simulink model "sanduan"  (R2018b)
settings: Solver=ode23s  StartTime=0.0  StopTime=2  RelTol=1e-3
libraries: powerlib_meascontrol x27, simulink_extras x27, powerlib x13
settings Model: Creator=snial  LastModifiedBy=snailtiny
settings DataIOCC: SaveFormat=StructureWithTime
settings OptimizationCC: LifeSpan=inf
settings DebuggingCC: SFExecutionAtInitializationDiag=none
settings HardwareCC: ProdBitPerSizeT=32  ProdBitPerPtrDiffT=32  ProdWordSize=32  ProdHWDeviceType=Specified
settings SFSimCC: SimUseLocalCustomCode=off
settings RTWCC: RTWUseLocalCustomCode=off
settings CodeAppCC: StateflowObjectComments=on
settings SimscapeCC: SimscapeNormalizeSystem=off

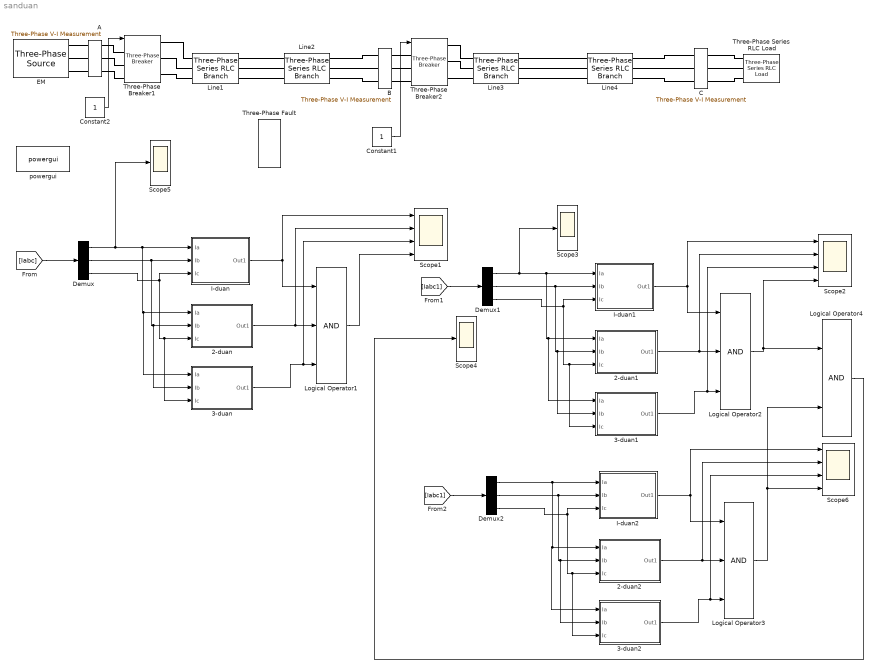
== system sanduan ==
  2-duan : Subsystem
  2-duan1 : Subsystem
  2-duan2 : Subsystem
  3-duan : Subsystem
  3-duan1 : Subsystem
  3-duan2 : Subsystem
  A : powerlib/Measurements/Three-Phase V-I Measurement  VoltageMeasurement=phase-to-ground  SetLabelV=on  LabelV=Vabc  Vpu=off  VpuLL=off  CurrentMeasurement=yes  SetLabelI=on  LabelI=Iabc  Ipu=off  Pbase=100e6  Vbase=500e3  OutputType=Complex  PhasorSimulation=off  PSBequivalent=0
      settings: SourceProductName=Simscape Electrical
  B : powerlib/Measurements/Three-Phase V-I Measurement  VoltageMeasurement=phase-to-ground  SetLabelV=on  LabelV=Vabc1  Vpu=off  VpuLL=off  CurrentMeasurement=yes  SetLabelI=on  LabelI=Iabc1  Ipu=off  Pbase=100e6  Vbase=500e3  OutputType=Complex  PhasorSimulation=off  PSBequivalent=0
      settings: SourceProductName=Simscape Electrical
  C : powerlib/Measurements/Three-Phase V-I Measurement  VoltageMeasurement=phase-to-ground  SetLabelV=on  LabelV=Vabc2  Vpu=off  VpuLL=off  CurrentMeasurement=yes  SetLabelI=on  LabelI=Iabc2  Ipu=off  Pbase=100e6  Vbase=500e3  OutputType=Complex  PhasorSimulation=off  PSBequivalent=0
      settings: SourceProductName=Simscape Electrical
  Constant1 : Constant
  Constant2 : Constant
  Demux : Demux  Outputs=3
  Demux1 : Demux  Outputs=3
  Demux2 : Demux  Outputs=3
  EM : powerlib/Electrical Sources/Three-Phase Source  InternalConnection=Yg  VoltagePhases=off  Voltage=37e3  PhaseAngle=0  Voltage_phases=[25e3 25e3 25e3]/sqrt(3)  PhaseAngles_phases=[0 -120 +120]  Frequency=50  NonIdealSource=on  SpecifyImpedance=off  Resistance=6  Inductance=0  ShortCircuitLevel=100e6  BaseVoltage=37e3  XRratio=7  BusType=swing  Pref=10e3  Qref=0  Prefabc=[10e3, 10e3, 10e3]  Qrefabc=[0, 0, 0]  Qmin=-inf  Qmax=inf
      settings: SourceProductName=Simscape Electrical
  I-duan : Subsystem
  I-duan1 : Subsystem
  I-duan2 : Subsystem
  Line1 : powerlib/Elements/Three-Phase Series RLC Branch  LConnTagsString=A|B|C  RConnTagsString=A|B|C  BranchType=R  Resistance=2  Inductance=0.00318*2  Capacitance=1e-6  Measurements=None
      settings: SourceProductName=Simscape Electrical
  Line2 : powerlib/Elements/Three-Phase Series RLC Branch  LConnTagsString=A|B|C  RConnTagsString=A|B|C  BranchType=R  Resistance=8  Inductance=0.00318*8  Capacitance=1e-6  Measurements=None
      settings: SourceProductName=Simscape Electrical
  Line3 : powerlib/Elements/Three-Phase Series RLC Branch  LConnTagsString=A|B|C  RConnTagsString=A|B|C  BranchType=R  Resistance=2  Inductance=0.00318*24  Capacitance=1e-6  Measurements=None
      settings: SourceProductName=Simscape Electrical
  Line4 : powerlib/Elements/Three-Phase Series RLC Branch  LConnTagsString=A|B|C  RConnTagsString=A|B|C  BranchType=R  Resistance=14  Inductance=0.00318*24  Capacitance=1e-6  Measurements=None
      settings: SourceProductName=Simscape Electrical
  Logical Operator1 : Logic  Inputs=3  AllPortsSameDT=off  OutDataTypeStr=boolean
  Logical Operator2 : Logic  Inputs=3  AllPortsSameDT=off  OutDataTypeStr=boolean
  Logical Operator3 : Logic  Inputs=3  AllPortsSameDT=off  OutDataTypeStr=boolean
  Logical Operator4 : Logic  AllPortsSameDT=off  OutDataTypeStr=boolean
  Scope1 : Scope  NumInputPorts=4
  Scope2 : Scope  NumInputPorts=4
  Scope3 : Scope
  Scope4 : Scope
  Scope5 : Scope
  Scope6 : Scope  NumInputPorts=4
  Three-Phase Series RLC Load : powerlib/Elements/Three-Phase Series RLC Load  LConnTagsString=A|B|C  Configuration=Y (grounded)  NominalVoltage=37e3  Vabc=[1e3 1e3 1e3]  Vabcp=[1e3 1e3 1e3]  NominalFrequency=50  UnbalancedPower=off  ActivePower=6.4e6  InductivePower=0  CapacitivePower=0  Pabc=[10e3 9e3 11e3]  QLabc=[100 90 110]  QCabc=[100 90 110]  Pabcp=[10e3 9e3 11e3]  QLabcp=[100 90 110]  QCabcp=[100 90 110]  Measurements=None  LoadType=constant Z
      settings: SourceProductName=Simscape Electrical
  Three-Phase Breaker1 : powerlib/Elements/Three-Phase Breaker  InitialState=closed  SwitchA=on  SwitchB=on  SwitchC=on  SwitchTimes="[1  1.20]"  External=on  BreakerResistance=0.0000000000000000001  SnubberResistance=1e6  SnubberCapacitance=inf  Measurements=None
      settings: SourceProductName=Simscape Electrical
  Three-Phase Breaker2 : powerlib/Elements/Three-Phase Breaker  InitialState=closed  SwitchA=on  SwitchB=on  SwitchC=on  SwitchTimes="[1  1.20]"  External=on  BreakerResistance=0.0000000000000000001  SnubberResistance=1e6  SnubberCapacitance=inf  Measurements=None
      settings: SourceProductName=Simscape Electrical
  Three-Phase Fault : powerlib/Elements/Three-Phase Fault  InitialStates=0  FaultA=on  FaultB=on  FaultC=off  GroundFault=off  SwitchTimes=[0.2 0.5]  External=off  SwitchStatus=NaN  FaultResistance=20  GroundResistance=0.01  SnubberResistance=inf  SnubberCapacitance=0  Measurements=None
      settings: SourceProductName=Simscape Electrical
  powergui : powerlib/powergui  Priority=1  SimulationMode=Continuous  SampleTime=1e-10  frequency=50  Iterations=50  frequencyindice=50  Pbase=100e6  ErrMax=1e-4  UnitsV=kV  UnitsW=MW  buscounter=0  FunctionMessages=off  echomessages=off  EnableUseOfTLC=off  CurrentSourceSwitches=off  DisableSnubberDevices=off  DisableRonSwitches=off  DisableVfSwitches=off  DisplayEquations=off  SolverType=Tustin/Backward Euler (TBE)  Interpol=off  ExternalGateDelay=off  methode=off  Ts=100  x0status=blocks  SPID=on  SwTol=0  HookPort=off  RestoreLinks=warning  ResistiveCurrentMeasurement=off  Frange=[0:2:500]  Ylog=off  Xlog=on  ShowGrid=off  save=off  variable=ZData  structure=0  ZoomFFT=off  StartTime=0.0  cycles=1  DisplayStyle=1  fundamental=60  FreqAxis=off  MaxFrequency=1000  frequencyindicesteady=1  RmsSteady=1  display=off
  wires:
  [Iabc] -> Demux/1
  Demux/1 -> Scope5/1, 3-duan/1(Ia), 2-duan/1(Ia), I-duan/1(Ia)
  Demux/2 -> 3-duan/2(Ib), 2-duan/2(Ib), I-duan/2(Ib)
  Demux/3 -> 3-duan/3(Ic), 2-duan/3(Ic), I-duan/3(Ic)
  I-duan/1(Out1) -> Scope1/1, Logical Operator1/1
  2-duan/1(Out1) -> Scope1/2, Logical Operator1/2
  3-duan/1(Out1) -> Scope1/3, Logical Operator1/3
  Logical Operator1/1 -> Scope1/4
  [Iabc1] -> Demux1/1
  Demux1/1 -> Scope3/1, 3-duan1/1(Ia), 2-duan1/1(Ia), I-duan1/1(Ia)
  Demux1/2 -> 3-duan1/2(Ib), 2-duan1/2(Ib), I-duan1/2(Ib)
  Demux1/3 -> 3-duan1/3(Ic), 2-duan1/3(Ic), I-duan1/3(Ic)
  I-duan1/1(Out1) -> Logical Operator2/1, Scope2/1
  2-duan1/1(Out1) -> Scope2/2, Logical Operator2/2
  3-duan1/1(Out1) -> Scope2/3, Logical Operator2/3
  Logical Operator2/1 -> Scope2/4, Logical Operator4/1
  Demux2/3 -> 3-duan2/3(Ic), 2-duan2/3(Ic), I-duan2/3(Ic)
  2-duan2/1(Out1) -> Scope6/2, Logical Operator3/2
  I-duan2/1(Out1) -> Scope6/1, Logical Operator3/1
  [Iabc1] -> Demux2/1
  Logical Operator3/1 -> Logical Operator4/2, Scope6/4
  Demux2/1 -> 3-duan2/1(Ia), 2-duan2/1(Ia), I-duan2/1(Ia)
  3-duan2/1(Out1) -> Scope6/3, Logical Operator3/3
  Demux2/2 -> 3-duan2/2(Ib), 2-duan2/2(Ib), I-duan2/2(Ib)
  Logical Operator4/1 -> Scope4/1
  Constant2/1 -> Three-Phase Breaker1/1
  Constant1/1 -> Three-Phase Breaker2/1
  connections:
  A/LConn1 -- EM/RConn1
  A/LConn2 -- EM/RConn2
  A/LConn3 -- EM/RConn3
  Line1/RConn2 -- Line2/LConn2
  Line1/RConn3 -- Line2/LConn3
  Line2/RConn1 -- B/LConn1
  Line2/RConn2 -- B/LConn2
  Line2/RConn3 -- B/LConn3
  C/RConn2 -- Three-Phase Series RLC Load/LConn2
  C/RConn3 -- Three-Phase Series RLC Load/LConn3
  C/RConn1 -- Three-Phase Series RLC Load/LConn1
  Three-Phase Breaker1/RConn1 -- Line1/LConn1
  Three-Phase Breaker1/RConn2 -- Line1/LConn2
  Three-Phase Breaker1/RConn3 -- Line1/LConn3
  Three-Phase Breaker1/LConn1 -- A/RConn1
  Three-Phase Breaker1/LConn2 -- A/RConn2
  Three-Phase Breaker1/LConn3 -- A/RConn3
  Line1/RConn1 -- Line2/LConn1
  Line4/LConn1 -- Line3/RConn1
  Line4/LConn3 -- Line3/RConn3
  Three-Phase Breaker2/LConn1 -- B/RConn1
  Three-Phase Breaker2/LConn2 -- B/RConn2
  Three-Phase Breaker2/LConn3 -- B/RConn3
  Three-Phase Breaker2/RConn1 -- Line3/LConn1
  Three-Phase Breaker2/RConn2 -- Line3/LConn2
  Three-Phase Breaker2/RConn3 -- Line3/LConn3
  Line4/RConn1 -- C/LConn1
  Line4/RConn2 -- C/LConn2
  Line4/RConn3 -- C/LConn3
  Line4/LConn2 -- Line3/RConn2

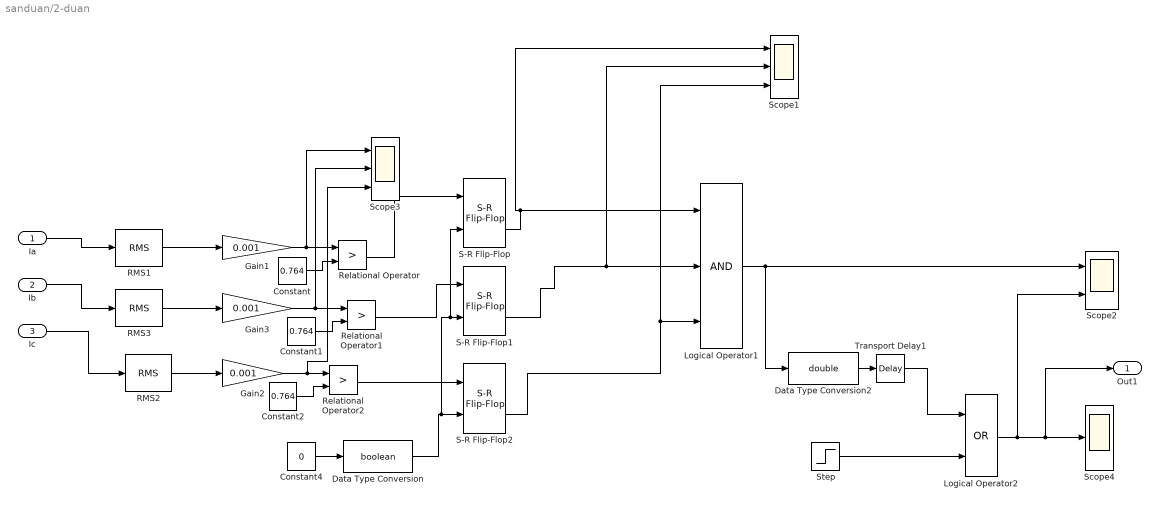
== system sanduan/2-duan ==
  Ia : Inport
  Ib : Inport  Port=2
  Ic : Inport  Port=3
  Constant : Constant  Value=0.764
  Constant1 : Constant  Value=0.764
  Constant2 : Constant  Value=0.764
  Constant4 : Constant  Value=0
  Data Type Conversion : DataTypeConversion  OutDataTypeStr=boolean
  Data Type Conversion2 : DataTypeConversion  OutDataTypeStr=double
  Gain1 : Gain  Gain=0.001
  Gain2 : Gain  Gain=0.001
  Gain3 : Gain  Gain=0.001
  Logical Operator1 : Logic  Inputs=3  AllPortsSameDT=off  OutDataTypeStr=boolean
  Logical Operator2 : Logic  Operator=OR  AllPortsSameDT=off  OutDataTypeStr=boolean
  RMS1 : powerlib_meascontrol/Measurements/RMS  TrueRMS=on  Freq=50  RMSInit=0  Ts=0
      settings: SourceProductName=Simscape Electrical
  RMS2 : powerlib_meascontrol/Measurements/RMS  TrueRMS=on  Freq=50  RMSInit=0  Ts=0
      settings: SourceProductName=Simscape Electrical
  RMS3 : powerlib_meascontrol/Measurements/RMS  TrueRMS=on  Freq=50  RMSInit=0  Ts=0
      settings: SourceProductName=Simscape Electrical
  Relational Operator : RelationalOperator  Operator=>  OutDataTypeStr=boolean  RndMeth=Nearest
  Relational Operator1 : RelationalOperator  Operator=>  OutDataTypeStr=boolean  RndMeth=Nearest
  Relational Operator2 : RelationalOperator  Operator=>  OutDataTypeStr=boolean  RndMeth=Nearest
  S-R Flip-Flop : simulink_extras/Flip Flops/S-R Flip-Flop  initial_condition=0
  S-R Flip-Flop1 : simulink_extras/Flip Flops/S-R Flip-Flop  initial_condition=0
  S-R Flip-Flop2 : simulink_extras/Flip Flops/S-R Flip-Flop  initial_condition=0
  Scope1 : Scope  NumInputPorts=3
  Scope2 : Scope  NumInputPorts=2
  Scope3 : Scope  NumInputPorts=3
  Scope4 : Scope
  Step : Step  Time=0.501  Before=1  After=0  SampleTime=0
  Transport Delay1 : TransportDelay  DelayTime=0.5
  Out1 : Outport
  wires:
  Ia/1 -> RMS1/1
  Constant/1 -> Relational Operator/2
  Gain1/1 -> Scope3/1, Relational Operator/1
  Constant1/1 -> Relational Operator1/2
  Gain3/1 -> Scope3/2, Relational Operator1/1
  Constant2/1 -> Relational Operator2/2
  Gain2/1 -> Scope3/3, Relational Operator2/1
  Relational Operator/1 -> S-R Flip-Flop/1
  Relational Operator1/1 -> S-R Flip-Flop1/1
  Relational Operator2/1 -> S-R Flip-Flop2/1
  Constant4/1 -> Data Type Conversion/1
  Data Type Conversion/1 -> S-R Flip-Flop/2, S-R Flip-Flop1/2, S-R Flip-Flop2/2
  RMS1/1 -> Gain1/1
  Ib/1 -> RMS3/1
  RMS3/1 -> Gain3/1
  Ic/1 -> RMS2/1
  RMS2/1 -> Gain2/1
  S-R Flip-Flop2/2 -> Scope1/3, Logical Operator1/3
  S-R Flip-Flop1/2 -> Scope1/2, Logical Operator1/2
  S-R Flip-Flop/2 -> Scope1/1, Logical Operator1/1
  Data Type Conversion2/1 -> Transport Delay1/1
  Logical Operator1/1 -> Scope2/1, Data Type Conversion2/1
  Transport Delay1/1 -> Logical Operator2/1
  Logical Operator2/1 -> Scope2/2, Out1/1, Scope4/1
  Step/1 -> Logical Operator2/2

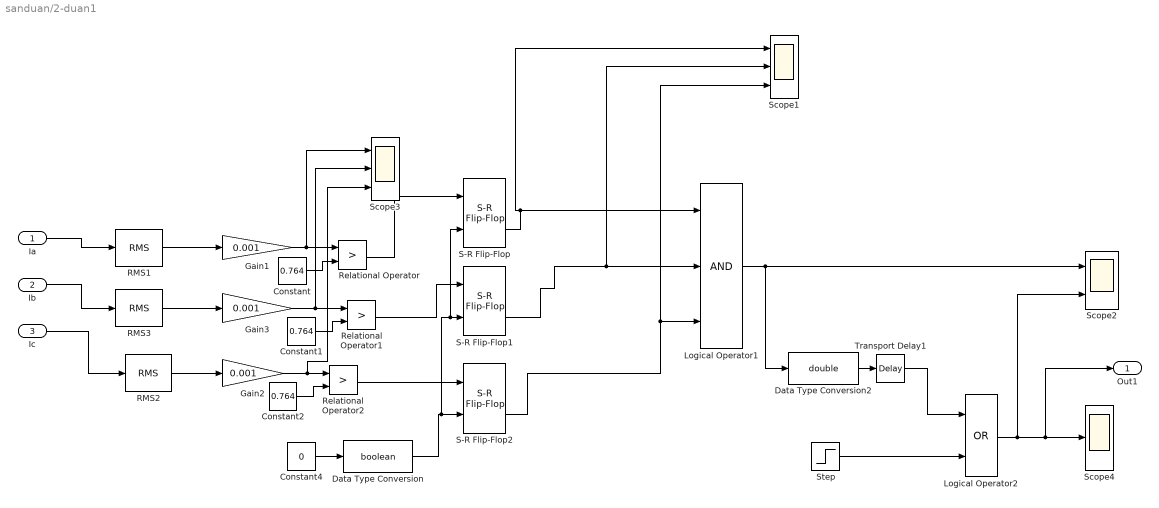
== system sanduan/2-duan1 ==
  Ia : Inport
  Ib : Inport  Port=2
  Ic : Inport  Port=3
  Constant : Constant  Value=0.764
  Constant1 : Constant  Value=0.764
  Constant2 : Constant  Value=0.764
  Constant4 : Constant  Value=0
  Data Type Conversion : DataTypeConversion  OutDataTypeStr=boolean
  Data Type Conversion2 : DataTypeConversion  OutDataTypeStr=double
  Gain1 : Gain  Gain=0.001
  Gain2 : Gain  Gain=0.001
  Gain3 : Gain  Gain=0.001
  Logical Operator1 : Logic  Inputs=3  AllPortsSameDT=off  OutDataTypeStr=boolean
  Logical Operator2 : Logic  Operator=OR  AllPortsSameDT=off  OutDataTypeStr=boolean
  RMS1 : powerlib_meascontrol/Measurements/RMS  TrueRMS=on  Freq=50  RMSInit=0  Ts=0
      settings: SourceProductName=Simscape Electrical
  RMS2 : powerlib_meascontrol/Measurements/RMS  TrueRMS=on  Freq=50  RMSInit=0  Ts=0
      settings: SourceProductName=Simscape Electrical
  RMS3 : powerlib_meascontrol/Measurements/RMS  TrueRMS=on  Freq=50  RMSInit=0  Ts=0
      settings: SourceProductName=Simscape Electrical
  Relational Operator : RelationalOperator  Operator=>  OutDataTypeStr=boolean  RndMeth=Nearest
  Relational Operator1 : RelationalOperator  Operator=>  OutDataTypeStr=boolean  RndMeth=Nearest
  Relational Operator2 : RelationalOperator  Operator=>  OutDataTypeStr=boolean  RndMeth=Nearest
  S-R Flip-Flop : simulink_extras/Flip Flops/S-R Flip-Flop  initial_condition=0
  S-R Flip-Flop1 : simulink_extras/Flip Flops/S-R Flip-Flop  initial_condition=0
  S-R Flip-Flop2 : simulink_extras/Flip Flops/S-R Flip-Flop  initial_condition=0
  Scope1 : Scope  NumInputPorts=3
  Scope2 : Scope  NumInputPorts=2
  Scope3 : Scope  NumInputPorts=3
  Scope4 : Scope
  Step : Step  Time=2  Before=1  After=0  SampleTime=0
  Transport Delay1 : TransportDelay  DelayTime=0.5
  Out1 : Outport
  wires:
  Ia/1 -> RMS1/1
  Constant/1 -> Relational Operator/2
  Gain1/1 -> Scope3/1, Relational Operator/1
  Constant1/1 -> Relational Operator1/2
  Gain3/1 -> Scope3/2, Relational Operator1/1
  Constant2/1 -> Relational Operator2/2
  Gain2/1 -> Scope3/3, Relational Operator2/1
  Relational Operator/1 -> S-R Flip-Flop/1
  Relational Operator1/1 -> S-R Flip-Flop1/1
  Relational Operator2/1 -> S-R Flip-Flop2/1
  Constant4/1 -> Data Type Conversion/1
  Data Type Conversion/1 -> S-R Flip-Flop/2, S-R Flip-Flop1/2, S-R Flip-Flop2/2
  RMS1/1 -> Gain1/1
  Ib/1 -> RMS3/1
  RMS3/1 -> Gain3/1
  Ic/1 -> RMS2/1
  RMS2/1 -> Gain2/1
  S-R Flip-Flop2/2 -> Scope1/3, Logical Operator1/3
  S-R Flip-Flop1/2 -> Scope1/2, Logical Operator1/2
  S-R Flip-Flop/2 -> Scope1/1, Logical Operator1/1
  Data Type Conversion2/1 -> Transport Delay1/1
  Logical Operator1/1 -> Scope2/1, Data Type Conversion2/1
  Transport Delay1/1 -> Logical Operator2/1
  Logical Operator2/1 -> Scope2/2, Out1/1, Scope4/1
  Step/1 -> Logical Operator2/2

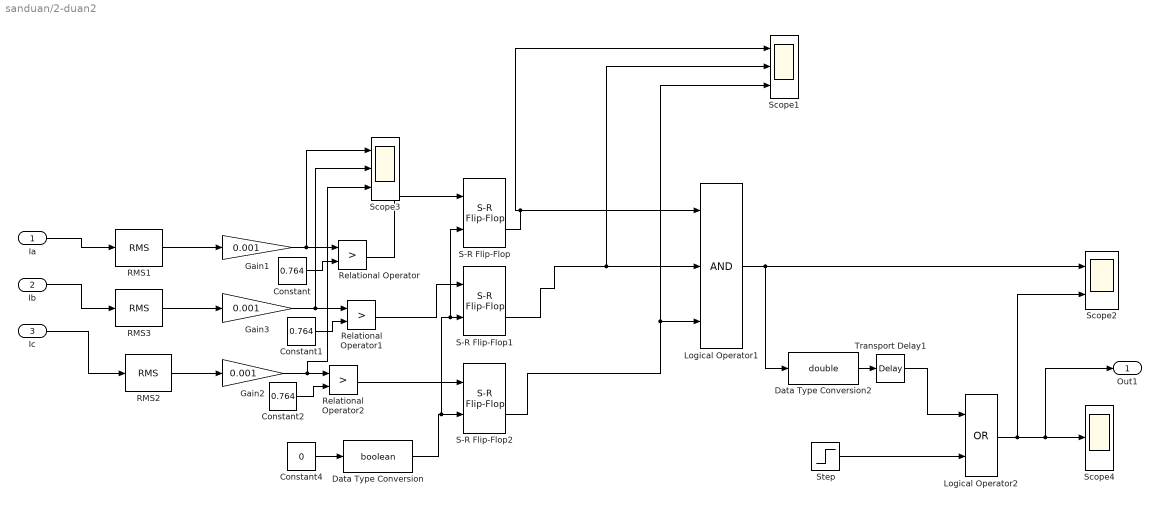
== system sanduan/2-duan2 ==
  Ia : Inport
  Ib : Inport  Port=2
  Ic : Inport  Port=3
  Constant : Constant  Value=0.764
  Constant1 : Constant  Value=0.764
  Constant2 : Constant  Value=0.764
  Constant4 : Constant  Value=0
  Data Type Conversion : DataTypeConversion  OutDataTypeStr=boolean
  Data Type Conversion2 : DataTypeConversion  OutDataTypeStr=double
  Gain1 : Gain  Gain=0.001
  Gain2 : Gain  Gain=0.001
  Gain3 : Gain  Gain=0.001
  Logical Operator1 : Logic  Inputs=3  AllPortsSameDT=off  OutDataTypeStr=boolean
  Logical Operator2 : Logic  Operator=OR  AllPortsSameDT=off  OutDataTypeStr=boolean
  RMS1 : powerlib_meascontrol/Measurements/RMS  TrueRMS=on  Freq=50  RMSInit=0  Ts=0
      settings: SourceProductName=Simscape Electrical
  RMS2 : powerlib_meascontrol/Measurements/RMS  TrueRMS=on  Freq=50  RMSInit=0  Ts=0
      settings: SourceProductName=Simscape Electrical
  RMS3 : powerlib_meascontrol/Measurements/RMS  TrueRMS=on  Freq=50  RMSInit=0  Ts=0
      settings: SourceProductName=Simscape Electrical
  Relational Operator : RelationalOperator  Operator=>  OutDataTypeStr=boolean  RndMeth=Nearest
  Relational Operator1 : RelationalOperator  Operator=>  OutDataTypeStr=boolean  RndMeth=Nearest
  Relational Operator2 : RelationalOperator  Operator=>  OutDataTypeStr=boolean  RndMeth=Nearest
  S-R Flip-Flop : simulink_extras/Flip Flops/S-R Flip-Flop  initial_condition=0
  S-R Flip-Flop1 : simulink_extras/Flip Flops/S-R Flip-Flop  initial_condition=0
  S-R Flip-Flop2 : simulink_extras/Flip Flops/S-R Flip-Flop  initial_condition=0
  Scope1 : Scope  NumInputPorts=3
  Scope2 : Scope  NumInputPorts=2
  Scope3 : Scope  NumInputPorts=3
  Scope4 : Scope
  Step : Step  Time=2  Before=1  After=0  SampleTime=0
  Transport Delay1 : TransportDelay  DelayTime=0.5
  Out1 : Outport
  wires:
  Ia/1 -> RMS1/1
  Constant/1 -> Relational Operator/2
  Gain1/1 -> Scope3/1, Relational Operator/1
  Constant1/1 -> Relational Operator1/2
  Gain3/1 -> Scope3/2, Relational Operator1/1
  Constant2/1 -> Relational Operator2/2
  Gain2/1 -> Scope3/3, Relational Operator2/1
  Relational Operator/1 -> S-R Flip-Flop/1
  Relational Operator1/1 -> S-R Flip-Flop1/1
  Relational Operator2/1 -> S-R Flip-Flop2/1
  Constant4/1 -> Data Type Conversion/1
  Data Type Conversion/1 -> S-R Flip-Flop/2, S-R Flip-Flop1/2, S-R Flip-Flop2/2
  RMS1/1 -> Gain1/1
  Ib/1 -> RMS3/1
  RMS3/1 -> Gain3/1
  Ic/1 -> RMS2/1
  RMS2/1 -> Gain2/1
  S-R Flip-Flop2/2 -> Scope1/3, Logical Operator1/3
  S-R Flip-Flop1/2 -> Scope1/2, Logical Operator1/2
  S-R Flip-Flop/2 -> Scope1/1, Logical Operator1/1
  Data Type Conversion2/1 -> Transport Delay1/1
  Logical Operator1/1 -> Scope2/1, Data Type Conversion2/1
  Transport Delay1/1 -> Logical Operator2/1
  Logical Operator2/1 -> Scope2/2, Out1/1, Scope4/1
  Step/1 -> Logical Operator2/2

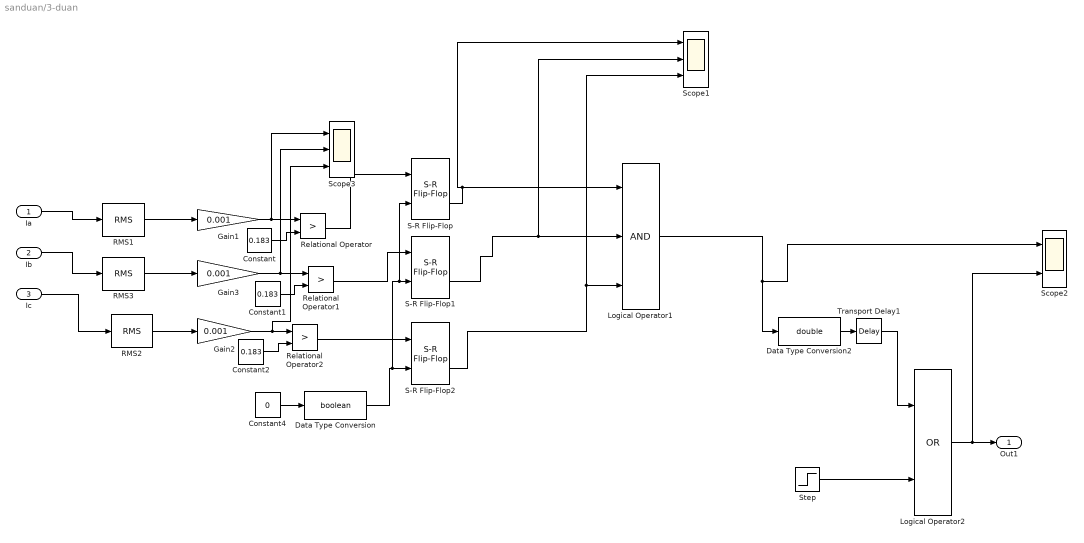
== system sanduan/3-duan ==
  Ia : Inport
  Ib : Inport  Port=2
  Ic : Inport  Port=3
  Constant : Constant  Value=0.183
  Constant1 : Constant  Value=0.183
  Constant2 : Constant  Value=0.183
  Constant4 : Constant  Value=0
  Data Type Conversion : DataTypeConversion  OutDataTypeStr=boolean
  Data Type Conversion2 : DataTypeConversion  OutDataTypeStr=double
  Gain1 : Gain  Gain=0.001
  Gain2 : Gain  Gain=0.001
  Gain3 : Gain  Gain=0.001
  Logical Operator1 : Logic  Inputs=3  AllPortsSameDT=off  OutDataTypeStr=boolean
  Logical Operator2 : Logic  Operator=OR  AllPortsSameDT=off  OutDataTypeStr=boolean
  RMS1 : powerlib_meascontrol/Measurements/RMS  TrueRMS=on  Freq=50  RMSInit=0  Ts=0
      settings: SourceProductName=Simscape Electrical
  RMS2 : powerlib_meascontrol/Measurements/RMS  TrueRMS=on  Freq=50  RMSInit=0  Ts=0
      settings: SourceProductName=Simscape Electrical
  RMS3 : powerlib_meascontrol/Measurements/RMS  TrueRMS=on  Freq=50  RMSInit=0  Ts=0
      settings: SourceProductName=Simscape Electrical
  Relational Operator : RelationalOperator  Operator=>  OutDataTypeStr=boolean  RndMeth=Nearest
  Relational Operator1 : RelationalOperator  Operator=>  OutDataTypeStr=boolean  RndMeth=Nearest
  Relational Operator2 : RelationalOperator  Operator=>  OutDataTypeStr=boolean  RndMeth=Nearest
  S-R Flip-Flop : simulink_extras/Flip Flops/S-R Flip-Flop  initial_condition=0
  S-R Flip-Flop1 : simulink_extras/Flip Flops/S-R Flip-Flop  initial_condition=0
  S-R Flip-Flop2 : simulink_extras/Flip Flops/S-R Flip-Flop  initial_condition=0
  Scope1 : Scope  NumInputPorts=3
  Scope2 : Scope  NumInputPorts=2
  Scope3 : Scope  NumInputPorts=3
  Step : Step  Time=1.501  Before=1  After=0  SampleTime=0
  Transport Delay1 : TransportDelay  DelayTime=1.5
  Out1 : Outport
  wires:
  Ia/1 -> RMS1/1
  Constant/1 -> Relational Operator/2
  Gain1/1 -> Scope3/1, Relational Operator/1
  Constant1/1 -> Relational Operator1/2
  Gain3/1 -> Scope3/2, Relational Operator1/1
  Constant2/1 -> Relational Operator2/2
  Gain2/1 -> Scope3/3, Relational Operator2/1
  Relational Operator/1 -> S-R Flip-Flop/1
  Relational Operator1/1 -> S-R Flip-Flop1/1
  Relational Operator2/1 -> S-R Flip-Flop2/1
  Constant4/1 -> Data Type Conversion/1
  Data Type Conversion/1 -> S-R Flip-Flop/2, S-R Flip-Flop1/2, S-R Flip-Flop2/2
  RMS1/1 -> Gain1/1
  Ib/1 -> RMS3/1
  RMS3/1 -> Gain3/1
  Ic/1 -> RMS2/1
  RMS2/1 -> Gain2/1
  Transport Delay1/1 -> Logical Operator2/1
  S-R Flip-Flop2/2 -> Scope1/3, Logical Operator1/3
  S-R Flip-Flop1/2 -> Scope1/2, Logical Operator1/2
  S-R Flip-Flop/2 -> Scope1/1, Logical Operator1/1
  Data Type Conversion2/1 -> Transport Delay1/1
  Logical Operator1/1 -> Scope2/1, Data Type Conversion2/1
  Step/1 -> Logical Operator2/2
  Logical Operator2/1 -> Scope2/2, Out1/1

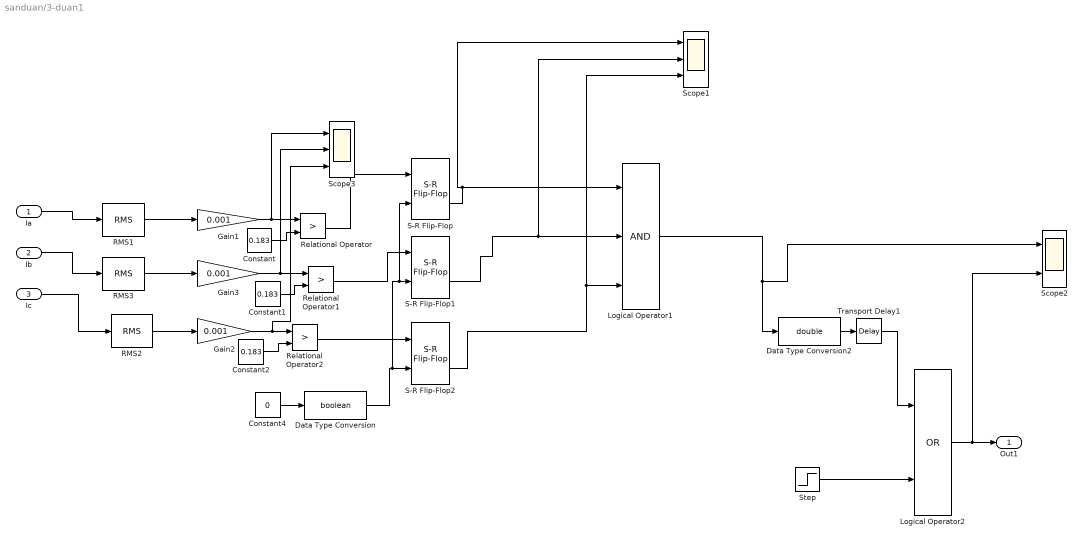
== system sanduan/3-duan1 ==
  Ia : Inport
  Ib : Inport  Port=2
  Ic : Inport  Port=3
  Constant : Constant  Value=0.183
  Constant1 : Constant  Value=0.183
  Constant2 : Constant  Value=0.183
  Constant4 : Constant  Value=0
  Data Type Conversion : DataTypeConversion  OutDataTypeStr=boolean
  Data Type Conversion2 : DataTypeConversion  OutDataTypeStr=double
  Gain1 : Gain  Gain=0.001
  Gain2 : Gain  Gain=0.001
  Gain3 : Gain  Gain=0.001
  Logical Operator1 : Logic  Inputs=3  AllPortsSameDT=off  OutDataTypeStr=boolean
  Logical Operator2 : Logic  Operator=OR  AllPortsSameDT=off  OutDataTypeStr=boolean
  RMS1 : powerlib_meascontrol/Measurements/RMS  TrueRMS=on  Freq=50  RMSInit=0  Ts=0
      settings: SourceProductName=Simscape Electrical
  RMS2 : powerlib_meascontrol/Measurements/RMS  TrueRMS=on  Freq=50  RMSInit=0  Ts=0
      settings: SourceProductName=Simscape Electrical
  RMS3 : powerlib_meascontrol/Measurements/RMS  TrueRMS=on  Freq=50  RMSInit=0  Ts=0
      settings: SourceProductName=Simscape Electrical
  Relational Operator : RelationalOperator  Operator=>  OutDataTypeStr=boolean  RndMeth=Nearest
  Relational Operator1 : RelationalOperator  Operator=>  OutDataTypeStr=boolean  RndMeth=Nearest
  Relational Operator2 : RelationalOperator  Operator=>  OutDataTypeStr=boolean  RndMeth=Nearest
  S-R Flip-Flop : simulink_extras/Flip Flops/S-R Flip-Flop  initial_condition=0
  S-R Flip-Flop1 : simulink_extras/Flip Flops/S-R Flip-Flop  initial_condition=0
  S-R Flip-Flop2 : simulink_extras/Flip Flops/S-R Flip-Flop  initial_condition=0
  Scope1 : Scope  NumInputPorts=3
  Scope2 : Scope  NumInputPorts=2
  Scope3 : Scope  NumInputPorts=3
  Step : Step  Time=2  Before=1  After=0  SampleTime=0
  Transport Delay1 : TransportDelay  DelayTime=1.5
  Out1 : Outport
  wires:
  Ia/1 -> RMS1/1
  Constant/1 -> Relational Operator/2
  Gain1/1 -> Scope3/1, Relational Operator/1
  Constant1/1 -> Relational Operator1/2
  Gain3/1 -> Scope3/2, Relational Operator1/1
  Constant2/1 -> Relational Operator2/2
  Gain2/1 -> Scope3/3, Relational Operator2/1
  Relational Operator/1 -> S-R Flip-Flop/1
  Relational Operator1/1 -> S-R Flip-Flop1/1
  Relational Operator2/1 -> S-R Flip-Flop2/1
  Constant4/1 -> Data Type Conversion/1
  Data Type Conversion/1 -> S-R Flip-Flop/2, S-R Flip-Flop1/2, S-R Flip-Flop2/2
  RMS1/1 -> Gain1/1
  Ib/1 -> RMS3/1
  RMS3/1 -> Gain3/1
  Ic/1 -> RMS2/1
  RMS2/1 -> Gain2/1
  Transport Delay1/1 -> Logical Operator2/1
  S-R Flip-Flop2/2 -> Scope1/3, Logical Operator1/3
  S-R Flip-Flop1/2 -> Scope1/2, Logical Operator1/2
  S-R Flip-Flop/2 -> Scope1/1, Logical Operator1/1
  Data Type Conversion2/1 -> Transport Delay1/1
  Logical Operator1/1 -> Scope2/1, Data Type Conversion2/1
  Step/1 -> Logical Operator2/2
  Logical Operator2/1 -> Scope2/2, Out1/1

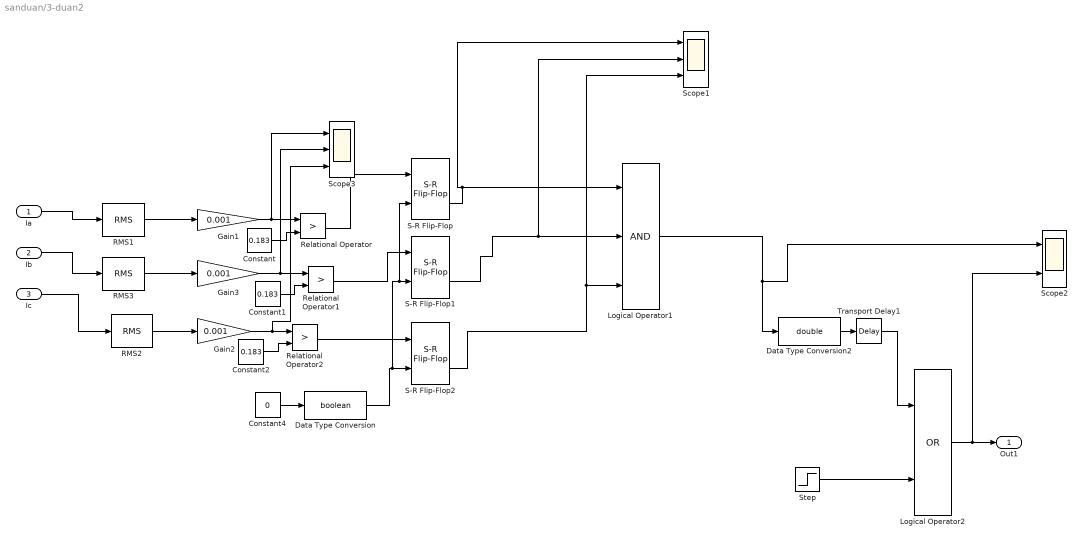
== system sanduan/3-duan2 ==
  Ia : Inport
  Ib : Inport  Port=2
  Ic : Inport  Port=3
  Constant : Constant  Value=0.183
  Constant1 : Constant  Value=0.183
  Constant2 : Constant  Value=0.183
  Constant4 : Constant  Value=0
  Data Type Conversion : DataTypeConversion  OutDataTypeStr=boolean
  Data Type Conversion2 : DataTypeConversion  OutDataTypeStr=double
  Gain1 : Gain  Gain=0.001
  Gain2 : Gain  Gain=0.001
  Gain3 : Gain  Gain=0.001
  Logical Operator1 : Logic  Inputs=3  AllPortsSameDT=off  OutDataTypeStr=boolean
  Logical Operator2 : Logic  Operator=OR  AllPortsSameDT=off  OutDataTypeStr=boolean
  RMS1 : powerlib_meascontrol/Measurements/RMS  TrueRMS=on  Freq=50  RMSInit=0  Ts=0
      settings: SourceProductName=Simscape Electrical
  RMS2 : powerlib_meascontrol/Measurements/RMS  TrueRMS=on  Freq=50  RMSInit=0  Ts=0
      settings: SourceProductName=Simscape Electrical
  RMS3 : powerlib_meascontrol/Measurements/RMS  TrueRMS=on  Freq=50  RMSInit=0  Ts=0
      settings: SourceProductName=Simscape Electrical
  Relational Operator : RelationalOperator  Operator=>  OutDataTypeStr=boolean  RndMeth=Nearest
  Relational Operator1 : RelationalOperator  Operator=>  OutDataTypeStr=boolean  RndMeth=Nearest
  Relational Operator2 : RelationalOperator  Operator=>  OutDataTypeStr=boolean  RndMeth=Nearest
  S-R Flip-Flop : simulink_extras/Flip Flops/S-R Flip-Flop  initial_condition=0
  S-R Flip-Flop1 : simulink_extras/Flip Flops/S-R Flip-Flop  initial_condition=0
  S-R Flip-Flop2 : simulink_extras/Flip Flops/S-R Flip-Flop  initial_condition=0
  Scope1 : Scope  NumInputPorts=3
  Scope2 : Scope  NumInputPorts=2
  Scope3 : Scope  NumInputPorts=3
  Step : Step  Time=2  Before=1  After=0  SampleTime=0
  Transport Delay1 : TransportDelay  DelayTime=1.5
  Out1 : Outport
  wires:
  Ia/1 -> RMS1/1
  Constant/1 -> Relational Operator/2
  Gain1/1 -> Scope3/1, Relational Operator/1
  Constant1/1 -> Relational Operator1/2
  Gain3/1 -> Scope3/2, Relational Operator1/1
  Constant2/1 -> Relational Operator2/2
  Gain2/1 -> Scope3/3, Relational Operator2/1
  Relational Operator/1 -> S-R Flip-Flop/1
  Relational Operator1/1 -> S-R Flip-Flop1/1
  Relational Operator2/1 -> S-R Flip-Flop2/1
  Constant4/1 -> Data Type Conversion/1
  Data Type Conversion/1 -> S-R Flip-Flop/2, S-R Flip-Flop1/2, S-R Flip-Flop2/2
  RMS1/1 -> Gain1/1
  Ib/1 -> RMS3/1
  RMS3/1 -> Gain3/1
  Ic/1 -> RMS2/1
  RMS2/1 -> Gain2/1
  Transport Delay1/1 -> Logical Operator2/1
  S-R Flip-Flop2/2 -> Scope1/3, Logical Operator1/3
  S-R Flip-Flop1/2 -> Scope1/2, Logical Operator1/2
  S-R Flip-Flop/2 -> Scope1/1, Logical Operator1/1
  Data Type Conversion2/1 -> Transport Delay1/1
  Logical Operator1/1 -> Scope2/1, Data Type Conversion2/1
  Step/1 -> Logical Operator2/2
  Logical Operator2/1 -> Scope2/2, Out1/1

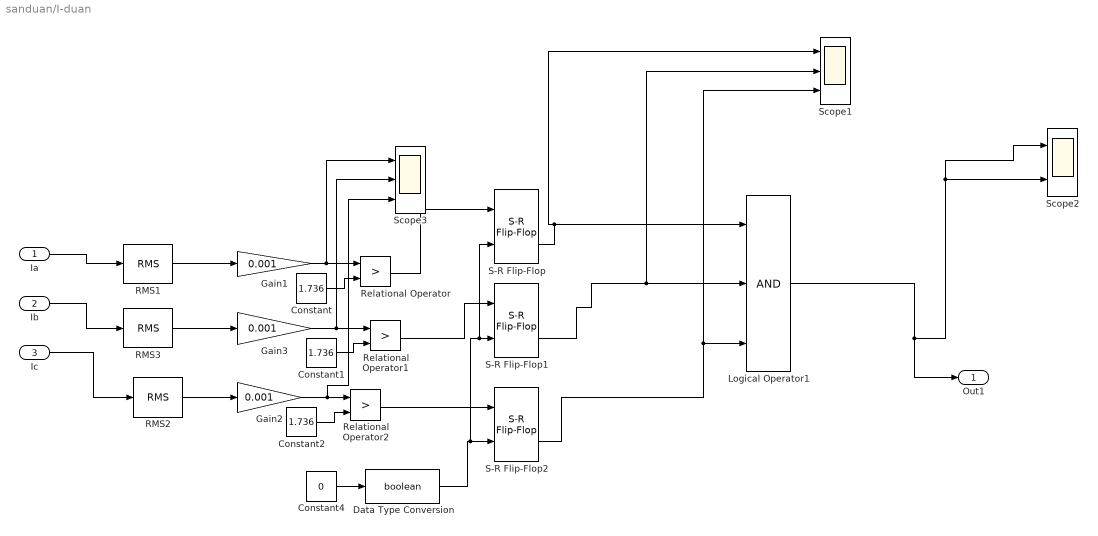
== system sanduan/I-duan ==
  Ia : Inport
  Ib : Inport  Port=2
  Ic : Inport  Port=3
  Constant : Constant  Value=1.736
  Constant1 : Constant  Value=1.736
  Constant2 : Constant  Value=1.736
  Constant4 : Constant  Value=0
  Data Type Conversion : DataTypeConversion  OutDataTypeStr=boolean
  Gain1 : Gain  Gain=0.001
  Gain2 : Gain  Gain=0.001
  Gain3 : Gain  Gain=0.001
  Logical Operator1 : Logic  Inputs=3  AllPortsSameDT=off  OutDataTypeStr=boolean
  RMS1 : powerlib_meascontrol/Measurements/RMS  TrueRMS=on  Freq=50  RMSInit=0  Ts=0
      settings: SourceProductName=Simscape Electrical
  RMS2 : powerlib_meascontrol/Measurements/RMS  TrueRMS=on  Freq=50  RMSInit=0  Ts=0
      settings: SourceProductName=Simscape Electrical
  RMS3 : powerlib_meascontrol/Measurements/RMS  TrueRMS=on  Freq=50  RMSInit=0  Ts=0
      settings: SourceProductName=Simscape Electrical
  Relational Operator : RelationalOperator  Operator=>  OutDataTypeStr=boolean  RndMeth=Nearest
  Relational Operator1 : RelationalOperator  Operator=>  OutDataTypeStr=boolean  RndMeth=Nearest
  Relational Operator2 : RelationalOperator  Operator=>  OutDataTypeStr=boolean  RndMeth=Nearest
  S-R Flip-Flop : simulink_extras/Flip Flops/S-R Flip-Flop  initial_condition=0
  S-R Flip-Flop1 : simulink_extras/Flip Flops/S-R Flip-Flop  initial_condition=0
  S-R Flip-Flop2 : simulink_extras/Flip Flops/S-R Flip-Flop  initial_condition=0
  Scope1 : Scope  NumInputPorts=3
  Scope2 : Scope  NumInputPorts=2
  Scope3 : Scope  NumInputPorts=3
  Out1 : Outport
  wires:
  Ia/1 -> RMS1/1
  Constant/1 -> Relational Operator/2
  Gain1/1 -> Scope3/1, Relational Operator/1
  Constant1/1 -> Relational Operator1/2
  Gain3/1 -> Scope3/2, Relational Operator1/1
  Constant2/1 -> Relational Operator2/2
  Gain2/1 -> Scope3/3, Relational Operator2/1
  Relational Operator/1 -> S-R Flip-Flop/1
  Relational Operator1/1 -> S-R Flip-Flop1/1
  Relational Operator2/1 -> S-R Flip-Flop2/1
  Constant4/1 -> Data Type Conversion/1
  Data Type Conversion/1 -> S-R Flip-Flop/2, S-R Flip-Flop1/2, S-R Flip-Flop2/2
  RMS1/1 -> Gain1/1
  Ib/1 -> RMS3/1
  RMS3/1 -> Gain3/1
  Ic/1 -> RMS2/1
  RMS2/1 -> Gain2/1
  S-R Flip-Flop2/2 -> Scope1/3, Logical Operator1/3
  S-R Flip-Flop1/2 -> Scope1/2, Logical Operator1/2
  S-R Flip-Flop/2 -> Scope1/1, Logical Operator1/1
  Logical Operator1/1 -> Scope2/2, Scope2/1, Out1/1

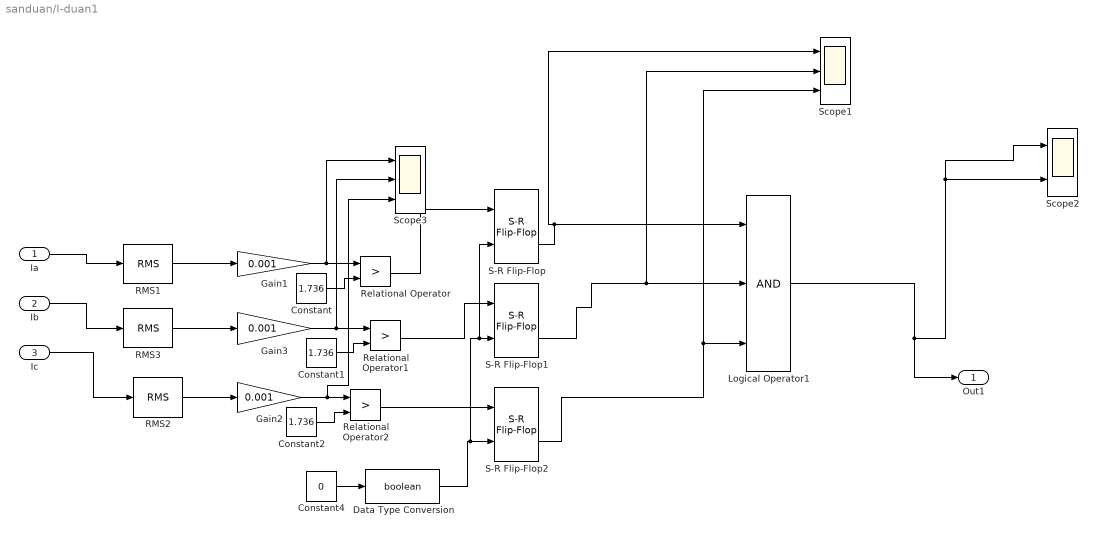
== system sanduan/I-duan1 ==
  Ia : Inport
  Ib : Inport  Port=2
  Ic : Inport  Port=3
  Constant : Constant  Value=1.736
  Constant1 : Constant  Value=1.736
  Constant2 : Constant  Value=1.736
  Constant4 : Constant  Value=0
  Data Type Conversion : DataTypeConversion  OutDataTypeStr=boolean
  Gain1 : Gain  Gain=0.001
  Gain2 : Gain  Gain=0.001
  Gain3 : Gain  Gain=0.001
  Logical Operator1 : Logic  Inputs=3  AllPortsSameDT=off  OutDataTypeStr=boolean
  RMS1 : powerlib_meascontrol/Measurements/RMS  TrueRMS=on  Freq=50  RMSInit=0  Ts=0
      settings: SourceProductName=Simscape Electrical
  RMS2 : powerlib_meascontrol/Measurements/RMS  TrueRMS=on  Freq=50  RMSInit=0  Ts=0
      settings: SourceProductName=Simscape Electrical
  RMS3 : powerlib_meascontrol/Measurements/RMS  TrueRMS=on  Freq=50  RMSInit=0  Ts=0
      settings: SourceProductName=Simscape Electrical
  Relational Operator : RelationalOperator  Operator=>  OutDataTypeStr=boolean  RndMeth=Nearest
  Relational Operator1 : RelationalOperator  Operator=>  OutDataTypeStr=boolean  RndMeth=Nearest
  Relational Operator2 : RelationalOperator  Operator=>  OutDataTypeStr=boolean  RndMeth=Nearest
  S-R Flip-Flop : simulink_extras/Flip Flops/S-R Flip-Flop  initial_condition=0
  S-R Flip-Flop1 : simulink_extras/Flip Flops/S-R Flip-Flop  initial_condition=0
  S-R Flip-Flop2 : simulink_extras/Flip Flops/S-R Flip-Flop  initial_condition=0
  Scope1 : Scope  NumInputPorts=3
  Scope2 : Scope  NumInputPorts=2
  Scope3 : Scope  NumInputPorts=3
  Out1 : Outport
  wires:
  Ia/1 -> RMS1/1
  Constant/1 -> Relational Operator/2
  Gain1/1 -> Scope3/1, Relational Operator/1
  Constant1/1 -> Relational Operator1/2
  Gain3/1 -> Scope3/2, Relational Operator1/1
  Constant2/1 -> Relational Operator2/2
  Gain2/1 -> Scope3/3, Relational Operator2/1
  Relational Operator/1 -> S-R Flip-Flop/1
  Relational Operator1/1 -> S-R Flip-Flop1/1
  Relational Operator2/1 -> S-R Flip-Flop2/1
  Constant4/1 -> Data Type Conversion/1
  Data Type Conversion/1 -> S-R Flip-Flop/2, S-R Flip-Flop1/2, S-R Flip-Flop2/2
  RMS1/1 -> Gain1/1
  Ib/1 -> RMS3/1
  RMS3/1 -> Gain3/1
  Ic/1 -> RMS2/1
  RMS2/1 -> Gain2/1
  S-R Flip-Flop2/2 -> Scope1/3, Logical Operator1/3
  S-R Flip-Flop1/2 -> Scope1/2, Logical Operator1/2
  S-R Flip-Flop/2 -> Scope1/1, Logical Operator1/1
  Logical Operator1/1 -> Scope2/2, Scope2/1, Out1/1

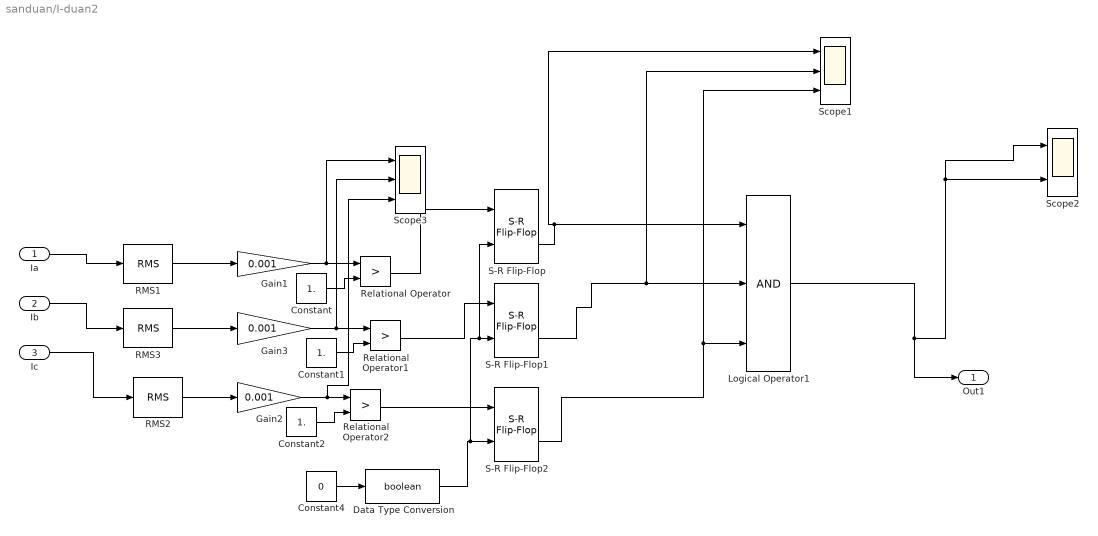
== system sanduan/I-duan2 ==
  Ia : Inport
  Ib : Inport  Port=2
  Ic : Inport  Port=3
  Constant : Constant  Value=1.
  Constant1 : Constant  Value=1.
  Constant2 : Constant  Value=1.
  Constant4 : Constant  Value=0
  Data Type Conversion : DataTypeConversion  OutDataTypeStr=boolean
  Gain1 : Gain  Gain=0.001
  Gain2 : Gain  Gain=0.001
  Gain3 : Gain  Gain=0.001
  Logical Operator1 : Logic  Inputs=3  AllPortsSameDT=off  OutDataTypeStr=boolean
  RMS1 : powerlib_meascontrol/Measurements/RMS  TrueRMS=on  Freq=50  RMSInit=0  Ts=0
      settings: SourceProductName=Simscape Electrical
  RMS2 : powerlib_meascontrol/Measurements/RMS  TrueRMS=on  Freq=50  RMSInit=0  Ts=0
      settings: SourceProductName=Simscape Electrical
  RMS3 : powerlib_meascontrol/Measurements/RMS  TrueRMS=on  Freq=50  RMSInit=0  Ts=0
      settings: SourceProductName=Simscape Electrical
  Relational Operator : RelationalOperator  Operator=>  OutDataTypeStr=boolean  RndMeth=Nearest
  Relational Operator1 : RelationalOperator  Operator=>  OutDataTypeStr=boolean  RndMeth=Nearest
  Relational Operator2 : RelationalOperator  Operator=>  OutDataTypeStr=boolean  RndMeth=Nearest
  S-R Flip-Flop : simulink_extras/Flip Flops/S-R Flip-Flop  initial_condition=0
  S-R Flip-Flop1 : simulink_extras/Flip Flops/S-R Flip-Flop  initial_condition=0
  S-R Flip-Flop2 : simulink_extras/Flip Flops/S-R Flip-Flop  initial_condition=0
  Scope1 : Scope  NumInputPorts=3
  Scope2 : Scope  NumInputPorts=2
  Scope3 : Scope  NumInputPorts=3
  Out1 : Outport
  wires:
  Ia/1 -> RMS1/1
  Constant/1 -> Relational Operator/2
  Gain1/1 -> Scope3/1, Relational Operator/1
  Constant1/1 -> Relational Operator1/2
  Gain3/1 -> Scope3/2, Relational Operator1/1
  Constant2/1 -> Relational Operator2/2
  Gain2/1 -> Scope3/3, Relational Operator2/1
  Relational Operator/1 -> S-R Flip-Flop/1
  Relational Operator1/1 -> S-R Flip-Flop1/1
  Relational Operator2/1 -> S-R Flip-Flop2/1
  Constant4/1 -> Data Type Conversion/1
  Data Type Conversion/1 -> S-R Flip-Flop/2, S-R Flip-Flop1/2, S-R Flip-Flop2/2
  RMS1/1 -> Gain1/1
  Ib/1 -> RMS3/1
  RMS3/1 -> Gain3/1
  Ic/1 -> RMS2/1
  RMS2/1 -> Gain2/1
  S-R Flip-Flop2/2 -> Scope1/3, Logical Operator1/3
  S-R Flip-Flop1/2 -> Scope1/2, Logical Operator1/2
  S-R Flip-Flop/2 -> Scope1/1, Logical Operator1/1
  Logical Operator1/1 -> Scope2/2, Scope2/1, Out1/1
